simulink model "L1_EX2"  (Simulink 6.0)
settings: Solver=ode45  StartTime=0.0  StopTime=10.0  RelTol=1e-3
undefined symbols (not defined in the file): kr
settings Model: LastModifiedBy=student

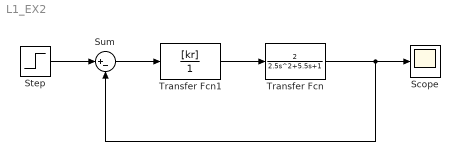
== system L1_EX2 ==
  Scope : Scope
  Step : Step  SampleTime=0
  Sum : Sum  Inputs=|+-
  Transfer Fcn : TransferFcn  Numerator=[2]  Denominator=[2.5 5.5 1]
  Transfer Fcn1 : TransferFcn  Numerator=[kr]  Denominator=[1]
  wires:
  Step/1 -> Sum/1
  Sum/1 -> Transfer Fcn1/1
  Transfer Fcn1/1 -> Transfer Fcn/1
  Transfer Fcn/1 -> Scope/1, Sum/2
